simulink model "vehicleDynamics"  (R2020a)
settings: Solver=VariableStepAuto  StartTime=0.0  StopTime=1588431736.7  RelTol=1e-3
model workspace (MAT data in the model file):
  SDO_OutputTimes = [1588431297.25 1588431297.3 1588431297.35 1588431297.4 1588431297.45 1588431297.5 1588431297.55 1588431297.6 1588431297.65 1588431297.7 1588431297.75 1588431297.8 ... (8790 elements, 8790x1)]
undefined symbols (not defined in the file): adc, g, KE, KT, L, m, magnitude, MFT, R, ra, rrc, vwc
(part 2 of 2)

== matlab function vehicleDynamics/ESC ==
  data: vin input; vout output; pedal input
function vout = fcn(vin, pedal)
vout = vin * pedal;
